simulink model "Crane1"  (Simulink 5.0)
settings: Solver=ode5  SolverMode=SingleTasking  StartTime=0.0  StopTime=50.0  FixedStep=0.001  RelTol=1e-3
libraries: pci1711 x3
settings Model: LastModifiedBy=AD  ExtModeMexFile=rtwinext  ExtModeTrigMode=oneshot  ExtModeTrigDuration=100000  ExtModeLogAll=off  SimulationMode=external  LimitDataPoints=off  BlockReductionOpt=off  BooleanDataType=off  RTWSystemTargetFile=rtwinfbk.tlc  RTWTemplateMakefile=winfbktmf  RTWOptions="-aCCOptimize=1 -aEnforceIntegerDowncast=1 -aExtMode=1 -aFoldNonRolledExpr=1 -aForceParamTrailComments=0 -aGenerateComments=1 -aGenerateReport=0 -aIncDataTypeInIds=0 -aIncHierarchyInIds=0 -aInlineInvariantSignals=0 -aInlineParameters=0 -aInlinedPrmAccess=\"Literals\" -aLocalBlockOutputs=1 -aMaxRTWIdLen=31 -aPrefixModelToSubsysFcnNames=1 -aRTWVerbose=1 -aRebuildAll=0 -aRollThreshold=5 -aShowEliminatedStatements=1"

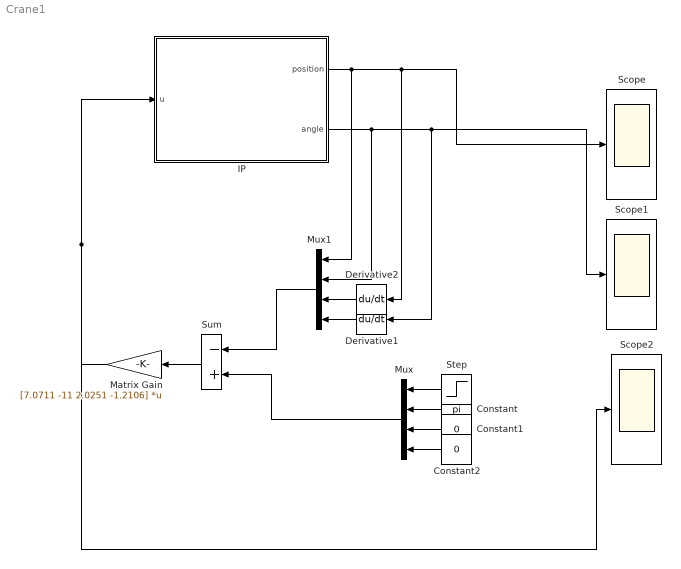
== system Crane1 ==
  Constant : Constant  Orientation=left  Value=pi
  Constant1 : Constant  Orientation=left  Value=0
  Constant2 : Constant  Orientation=left  Value=0
  Derivative1 : Derivative  Orientation=left
  Derivative2 : Derivative  Orientation=left
  IP : Subsystem
  Matrix Gain : Gain  Orientation=left  Gain=[7.0711 -11 2.0251 -1.2106]  Multiplication=Matrix(K*u)  SaturateOnIntegerOverflow=on
  Mux : Mux  Orientation=left
  Mux1 : Mux  Orientation=left
  Scope : Scope
      settings: TickLabels=on  TimeRange=50  YMin=-0.025  YMax=0.225  SaveName=y  SampleTime=0.01
  Scope1 : Scope
      settings: TickLabels=on  TimeRange=50  YMin=-0.025  YMax=0.225  SaveName=y1  SampleTime=0.01
  Scope2 : Scope
      settings: TickLabels=on  TimeRange=50  YMin=-0.025  YMax=0.225  SaveName=y2  SampleTime=0.01
  Step : Step  Orientation=left  Time=10  After=0.2  SampleTime=0
  Sum : Sum  Orientation=left  Inputs=-+  SaturateOnIntegerOverflow=on
  wires:
  IP/1(position) -> Derivative2/1, Scope/1, Mux1/1
  Matrix Gain/1 -> IP/1(u), Scope2/1
  Step/1 -> Mux/1
  Constant1/1 -> Mux/3
  Mux1/1 -> Sum/1
  Mux/1 -> Sum/2
  Derivative1/1 -> Mux1/4
  Derivative2/1 -> Mux1/3
  Sum/1 -> Matrix Gain/1
  IP/2(angle) -> Mux1/2, Scope1/1, Derivative1/1
  Constant/1 -> Mux/2
  Constant2/1 -> Mux/4

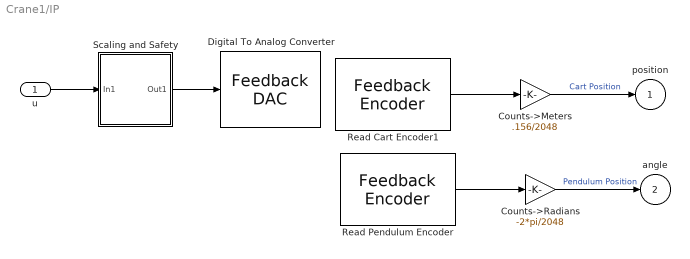
== system Crane1/IP ==
  u : Inport
  Counts->Meters : Gain  Gain=.156/2048  SaturateOnIntegerOverflow=on
  Counts->Radians : Gain  Gain=-2*pi/2048  SaturateOnIntegerOverflow=on
  Digital To Analog Converter : pci1711/Advantech  PCI1711 I//O Board Lib/Feedback DAC  channel=0  range=0  tsamp=0.001  hwAccess=on
  Read Cart Encoder1 : pci1711/Advantech  PCI1711 I//O Board Lib/Feedback Encoder   channel=0  offset=0  tsamp=0.001  hwAccess=on
  Read Pendulum Encoder : pci1711/Advantech  PCI1711 I//O Board Lib/Feedback Encoder   channel=1  offset=-1024  tsamp=0.001  hwAccess=on
  Scaling and Safety : Subsystem
  position : Outport
  angle : Outport  Port=2
  wires:
  Scaling and Safety/1(Out1) -> Digital To Analog Converter/1
  u/1 -> Scaling and Safety/1(In1)
  Read Cart Encoder1/1 -> Counts->Meters/1
  Read Pendulum Encoder/1 -> Counts->Radians/1
  Counts->Radians/1 -> angle/1  "Pendulum Position"
  Counts->Meters/1 -> position/1  "Cart Position"

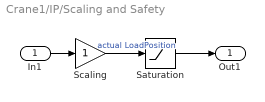
== system Crane1/IP/Scaling and Safety ==
  In1 : Inport
  Saturation : Saturate  UpperLimit=2.5  LowerLimit=-2.5
  Scaling : Gain  SaturateOnIntegerOverflow=on
  Out1 : Outport
  wires:
  Scaling/1 -> Saturation/1  "actual LoadPosition"
  In1/1 -> Scaling/1
  Saturation/1 -> Out1/1
